simulink model "AD_model"  (R2025b)
settings: Solver=VariableStepAuto  StartTime=0.0  StopTime=tspan  RelTol=1e-3
values from neighbouring files (symbols this model uses):
  activado = 0    [run_AD_F.m]    (also in run_AD_s.m; run_AD_s_control.m)
  C_CO20 = 9    [AnaerobicDigestorParameters.m]
  C_CO2Din = 0    [AnaerobicDigestorParameters.m]
  C_HCO3in = 0    [AnaerobicDigestorParameters.m]
  F1 = 1    [run_AD_F.m]    (also in run_AD_s.m; run_AD_s_control.m)
  F2 = F2jumps(i)    [run_AD_F.m]    (also in run_AD_s.m = 1; run_AD_s_control.m = 1)
  K1 = 6.5e-7    (= 6.5e-07)    [AnaerobicDigestorParameters.m]
  KH = 3.25e-2    (= 0.0325)    [AnaerobicDigestorParameters.m]
  Ki = 0.667    [AnaerobicDigestorParameters.m]
  kLa = 100    [AnaerobicDigestorParameters.m]
  Ks = 0.0333    [AnaerobicDigestorParameters.m]
  mumax = 0.4    [AnaerobicDigestorParameters.m]
  P = 760    [AnaerobicDigestorParameters.m]
  P_CO20 = 273    [AnaerobicDigestorParameters.m]
  pHoff = 7    [AnaerobicDigestorParameters.m]
  pHth1 = 6.75    [AnaerobicDigestorParameters.m]
  pHth2 = 6.65    [AnaerobicDigestorParameters.m]
  pKa = 4.5    [AnaerobicDigestorParameters.m]
  QR1 = 50    [AnaerobicDigestorParameters.m]
  QR2 = 175    [AnaerobicDigestorParameters.m]
  rhoG = 38.9    [AnaerobicDigestorParameters.m]
  s0 = 2    [AnaerobicDigestorParameters.m]
  sif1 = 167    [run_AD_F.m]    (also in run_AD_s.m; run_AD_s_control.m)
  sif2 = sif1    (= 167)    [run_AD_F.m]    (also in run_AD_s.m = sifjumps(2); run_AD_s_control.m = sifjumps(i))
  V = 10    [AnaerobicDigestorParameters.m]
  VG = 2.0    (= 2)    [AnaerobicDigestorParameters.m]
  x0 = 5.28    [AnaerobicDigestorParameters.m]
  xin = 0    [AnaerobicDigestorParameters.m]
  Ych4x = 28.8    [AnaerobicDigestorParameters.m]
  Yco2x = 28.8    [AnaerobicDigestorParameters.m]
  Yxs = 0.032    [AnaerobicDigestorParameters.m]
  z0 = 50    [AnaerobicDigestorParameters.m]
  zin = 50    [AnaerobicDigestorParameters.m]
settings Model: Creator=Rodolfo  LastModifiedBy=Rodolfo

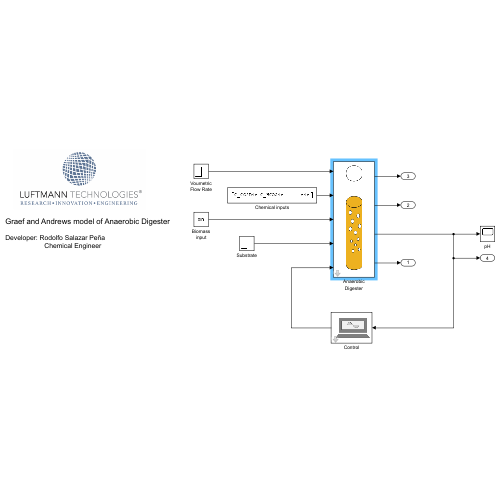
[thumbnail: Simulink's stored preview of the top-level diagram]
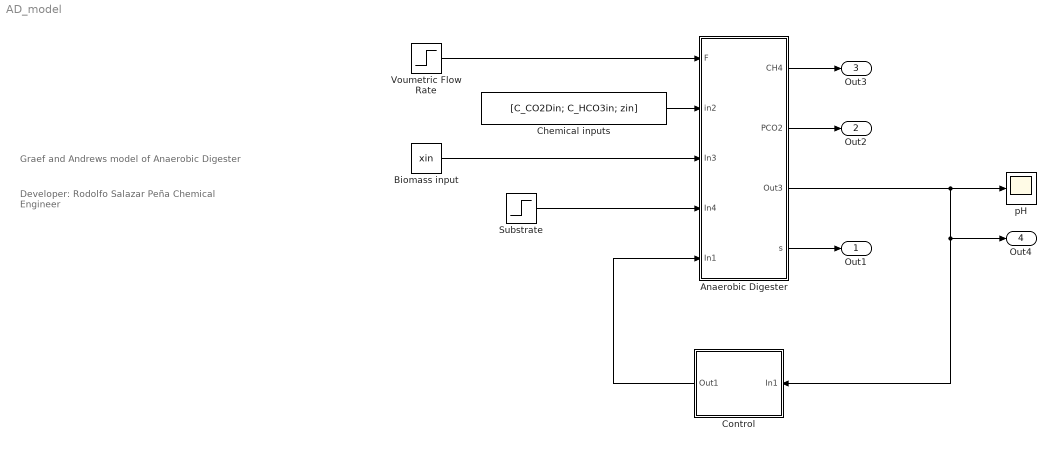
== system AD_model ==
  note: Developer: Rodolfo Salazar Peña
      | Chemical Engineer
  note: Graef and Andrews model of Anaerobic Digester
  Anaerobic Digester : Subsystem  mask(Anerobic Digester){VolumeParameter=V}
      mask prompts: VolumeParameter "Anarobic Digestor Volume"
      mask help: Integrated anaerobic digester model based on Graef and Andrews, combining biological, liquid, and gas phases for simulation and pH-oriented control studies.
      mask Help: This masked subsystem represents a complete anaerobic digester based on the Graef and Andrews model, integrating the biological, liquid, and gas phases into a unified dynamic framework. The biological phase describes the interaction between a generalized biomass and substrate using Haldane-type kinetics, accounting for substrate inhibition and biogas generation. The liquid phase models dissolved carbon dioxide and volatile fatty acids through chemical equilibria and gas–liquid mass transfer processes, enabling the determination and monitoring of pH to assess process stability and prevent acidification. The gas phase represents biogas release and composition, mainly methane and carbon dioxide, together with water vapor, hydrogen, and trace compounds, and supports control strategies based on gas manipulation, including the injection of inert compounds. This integrated model is intended for simulation, analysis, and control-oriented studies of anaerobic digestion systems.
  Biomass input : Constant  Value=xin
  Chemical inputs : Constant  Value=[C_CO2Din; C_HCO3in; zin]
  Control : Subsystem  mask(Control System){pHThreshold1=pHth1, pHThreshold2=pHth2, pHTurnedOff=pHoff, GasFlow1=QR1, GasFlow2=QR2}
      mask prompts: pHThreshold1 "pH Threshold 1"; pHThreshold2 "pH Threshold 2"; pHTurnedOff "pH off"; GasFlow1 "Volumetric Gas Flow Rate 1"; GasFlow2 "Volumetric Gas Flow Rate 2"
      mask help: Implements a two-stage relay control strategy based on pH monitoring to activate gas pumping and prevent acidification.
      mask Help: This masked subsystem implements a pH-based control strategy for the anaerobic digester. The pH of the liquid phase is continuously monitored and used as the controlled variable. Two relay elements with different threshold values define a staged control action. When the first pH threshold is reached, the first relay is activated, initiating gas pumping to mitigate acidification. If this action is insufficient and the pH continues to decrease until the second threshold is reached, a second relay is activated to increase the gas pumping rate. Once the pH returns to a neutral range, the activated pumps are deactivated. This subsystem is intended for dynamic simulation and evaluation of gas-based control strategies for acidification prevention.
      mask DialogControl pHParameterGroupVar Prompt: pH settings
      mask DialogControl GasFlows Prompt: Gas flow rates
  Substrate : Step  Before=sif1  After=sif2  SampleTime=0
  Voumetric Flow Rate : Step  Before=F1  After=F2  SampleTime=0
  pH : Scope
      settings: ActiveDisplayYMinimum=3.560384025804944  ActiveDisplayYMaximum=7.2867188541254588
  Out1 : Outport
  Out2 : Outport  Port=2
  Out3 : Outport  Port=3
  Out4 : Outport  Port=4
  wires:
  Chemical inputs/1 -> Anaerobic Digester/2(in2)
  Biomass input/1 -> Anaerobic Digester/3(In3)
  Substrate/1 -> Anaerobic Digester/4(In4)
  Anaerobic Digester/1(CH4) -> Out3/1
  Anaerobic Digester/2(PCO2) -> Out2/1
  Anaerobic Digester/4(s) -> Out1/1
  Anaerobic Digester/3(Out3) -> Control/1(In1), Out4/1, pH/1
  Voumetric Flow Rate/1 -> Anaerobic Digester/1(F)
  Control/1(Out1) -> Anaerobic Digester/5(In1)

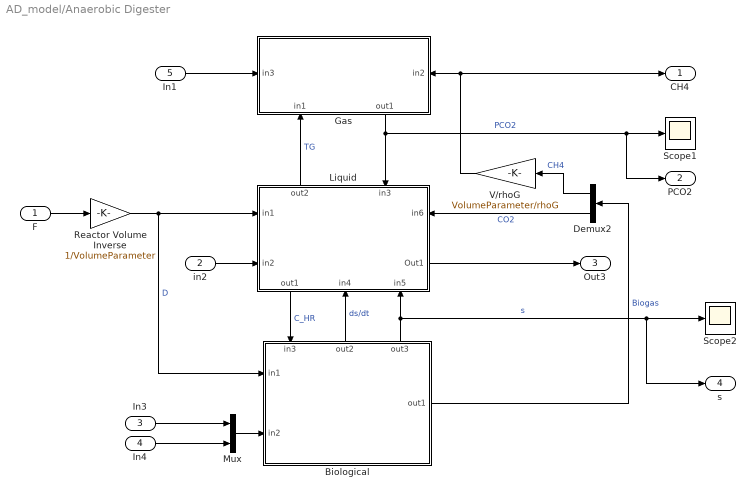
== system AD_model/Anaerobic Digester ==
  F : Inport
  in2 : Inport  Port=2
  In3 : Inport  Port=3
  In4 : Inport  Port=4
  In1 : Inport  Port=5
  Biological : Subsystem  Description=Image Credit: “Colorful Microorganisms: A Fascinating World Revealed” — image generated by Easy-Peasy.AI, licensed under Creative Commons. Source: easy-peasy.ai (https://easy-peasy.ai/ai-image-generator/images/colorful-microorganisms-intricate-shapes-forms-microbial-world  mask(Biological Phase){KinParameter1=mumax, KinParameter2=Ks, KinParameter3=Ki, YXS=Yxs, YCH4X=Ych4x, YCO2X=Yco2x, initx=x0, inits=s0}
      mask prompts: KinParameter1 "mu_max"; KinParameter2 "Ks"; KinParameter3 "Ki"; YXS "Y_x/s"; YCH4X "Y_CH4/x"; YCO2X "Y_CO2/x"; initx "x_0"; inits "s_0"
      mask help: Models the biological phase of an anaerobic digester with generalized biomass and substrate, using Haldane kinetics and biogas production (CH_4, CO_2).
      settings: PortSchema="{\"entries\":[{\"content\":{\"sides\":[{\"content\":{\"connectorIds\":[\"In1\",\"In2\"]},\"type\":\"ConnectorPlacement.EquallySpacedRectSide\",\"uuid\":\"94ecfc72-442c-41e1-8615-bec035df41b7\"},{\"content\":{\"connectorIds\":[\"Out1\"],\"side\":\"RIGHT\"},\"type\":\"ConnectorPlacement.EquallySpacedRectSide\",\"uuid\":\"bdca07f7-8c82-4860-9473-7970328f5f38\"},{\"content\":{\"connectorIds\":[\"In3\",\"Out2\",\"Out3\"],\"side\":\"TOP\"},\"type\":\"ConnectorPlacement.EquallySpacedRectSide\",\"uuid\":\"75f8fbf8-3bf9-45f3-a218-a686b6add209\"}]},\"type\":\"ConnectorPlacement.EquallySpacedConnector\",\"uuid\":\"e7f3f234-c871-423f-9938-c4e26176119c\"}],\"packageUris\":[\"http://schema.mathworks.com/mf0/Connector/R2020b\"],\"version\":\"1.0\"}"
      mask Help: This subsystem represents the biological phase of an anaerobic digester, describing the interaction between a generalized biomass 𝑥 and a substrate 𝑠. Microbial growth and substrate consumption are modeled using Haldane-type kinetics to account for substrate inhibition at high concentrations. Biogas production is computed as a consequence of the biological conversion process, with methane (CH_4) and carbon dioxide (CO_2) considered as the main gaseous products. The subsystem is intended for dynamic simulation and control-oriented analysis of anaerobic digestion processes.
      mask DialogControl KinParameterGroupVar Prompt: Kinetic Parameters
      mask DialogControl YieldsParameterGroupVar Prompt: Yields
      mask DialogControl InitialBio Prompt: Initial Conditions for Biological Phase
  Demux2 : Demux  Outputs=2
  Gas : Subsystem  Description=Image Credit: “Particle Model of a Gas (Teilchenmodell Gas)” — by Kaneiderdaniel, licensed under CC BY-SA 3.0. Source: Wikimedia Commons (File:Teilchenmodell_Gas.svg)  mask(Gas Phase){GasParameter1=P, GasParameter2=VG, GasParameter3=rhoG, InitGas=P_CO20}
      mask prompts: GasParameter1 "Pressure"; GasParameter2 "Gas Volume"; GasParameter3 "Gas Molar Density"; InitGas "CO2 Initial Partial Pressure"
      mask help: Models the gas phase of an anaerobic digester, including biogas release, composition dynamics, and gas-based control strategies to prevent acidification.
      settings: PortSchema="{\"entries\":[{\"content\":{\"sides\":[{\"content\":{\"connectorIds\":[\"In1\"]},\"type\":\"ConnectorPlacement.EquallySpacedRectSide\",\"uuid\":\"3565c727-b36c-46d2-95bd-ab32174b37cb\"},{\"content\":{\"connectorIds\":[\"In3\"],\"side\":\"RIGHT\"},\"type\":\"ConnectorPlacement.EquallySpacedRectSide\",\"uuid\":\"c4e665d1-7db3-4509-b4b2-58bd1ad74d47\"},{\"content\":{\"side\":\"TOP\"},\"type\":\"ConnectorPlacement.EquallySpacedRectSide\",\"uuid\":\"7f169c89-e67a-49df-a15c-98b353f69781\"},{\"content\":{\"connectorIds\":[\"In2\",\"Out1\"],\"side\":\"BOTTOM\"},\"type\":\"ConnectorPlacement.EquallySpacedRectSide\",\"uuid\":\"61ad4f32-0a2a-4148-a498-3c1351082a85\"}]},\"type\":\"ConnectorPlacement.EquallySpacedConnector\",\"uuid\":\"c5dc36fd-dcdd-47be-95df-e8a0ac72026a\"}],\"packageUris\":[\"http://schema.mathworks.com/mf0/Connector/R2020b\"],\"version\":\"1.0\"}"
      mask Help: This masked subsystem represents the gas phase of an anaerobic digester, where biogas is released as a result of biological conversion processes. The biogas is composed mainly of methane and carbon dioxide, along with water vapor, molecular hydrogen and trace compounds. The gas phase plays a key role in process operation and control, since acidification prevention strategies may involve the injection or removal of inert gases to influence gas composition, partial pressures, and gas–liquid equilibria. This subsystem is intended for dynamic simulation and control-oriented analysis of the anaerobic digestion process.
      mask DialogControl GasParameterGroupVar Prompt: Gas Parameters
      mask DialogControl GasInit Prompt: Gas Initial Conditions
  Liquid : Subsystem  Description=Image Credit: “Liquid Water Waves Background” — image by Andrea Stöckel, in the public domain (CC0). Source: PublicDomainPictures.net (https://www.publicdomainpictures.net/es/view-image.php?image=431076&picture=liquido-de-fondo-de-agua-de-ondas)  mask(Liquid phase of an anaerobic digester){TGParameter1=KH, TGParameter2=kLa, IonParameter1=pKa, IonParameter2=K1, InitLiquid1=C_CO20, InitLiquid2=z0}
      mask prompts: TGParameter1 "Henry's Law constant"; TGParameter2 "Bulk - Interphase constnat"; IonParameter1 "VFA Dissociation"; IonParameter2 "Dissolved CO2 Equilibrium"; InitLiquid1 "Dissolved CO2 Initial Concentration"; InitLiquid2 "Net Cationic Initial Concentration"
      mask help: Models liquid-phase chemistry and mass transfer in an anaerobic digester to compute and monitor pH and prevent acidification.
      settings: PortSchema="{\"entries\":[{\"content\":{\"sides\":[{\"content\":{\"connectorIds\":[\"In1\",\"In2\"]},\"type\":\"ConnectorPlacement.EquallySpacedRectSide\",\"uuid\":\"2cd52875-f219-461b-bc38-0fc8a9bb25f3\"},{\"content\":{\"connectorIds\":[\"In6\",\"Out1\"],\"side\":\"RIGHT\"},\"type\":\"ConnectorPlacement.EquallySpacedRectSide\",\"uuid\":\"4617526c-ef4d-41e9-b20c-a88def61ea23\"},{\"content\":{\"connectorIds\":[\"Out3\",\"In3\"],\"side\":\"TOP\"},\"type\":\"ConnectorPlacement.EquallySpacedRectSide\",\"uuid\":\"65a01b26-7f6a-43a7-a50c-408a5bf6dc68\"},{\"content\":{\"connectorIds\":[\"Out2\",\"In4\",\"In5\"],\"side\":\"BOTTOM\"},\"type\":\"ConnectorPlacement.EquallySpacedRectSide\",\"uuid\":\"34e478b9-109e-4b95-ae18-09426b257fdc\"}]},\"type\":\"ConnectorPlacement.EquallySpacedConnector\",\"uuid\":\"457643e1-ae11-400d-8d76-b246d90ceafd\"}],\"packageUris\":[\"http://schema.mathworks.com/mf0/Connector/R2020b\"],\"version\":\"1.0\"}"
      mask Help: This masked subsystem represents the liquid phase of an anaerobic digester, where dissolved carbon dioxide and volatile fatty acids (VFAs) undergo chemical equilibria and mass transfer processes. The model accounts for acid–base reactions, dissociation phenomena, and gas–liquid mass transfer effects that influence the hydrogen ion concentration. The primary objective of this subsystem is to determine and monitor the pH of the liquid phase in order to assess process stability and prevent acidification during anaerobic digestion.
      mask DialogControl TransferParameterGroupVar Prompt: Transfer CO2 gas - liquid
      mask DialogControl IonicParameters Prompt: Ionics Equilibriums
      mask DialogControl InitiLiquid Prompt: Initial Conditions for Liquid Phase
  Mux : Mux  Inputs=2
  Reactor Volume Inverse : Gain  Gain=1/VolumeParameter
  Scope1 : Scope
      settings: ActiveDisplayYMinimum=-1  ActiveDisplayYMaximum=1
  Scope2 : Scope
      settings: ActiveDisplayYMinimum=-1  ActiveDisplayYMaximum=1  DataLoggingVariableName=ScopeData2
  V/rhoG : Gain  Gain=VolumeParameter/rhoG
  CH4 : Outport
  PCO2 : Outport  Port=2
  Out3 : Outport  Port=3
  s : Outport  Port=4
  wires:
  Biological/2(out2) -> Liquid/4(in4)  "ds/dt"
  Liquid/2(out1) -> Biological/3(in3)  "C_HR"
  Liquid/3(out2) -> Gas/2(in1)  "TG"
  Biological/1(out1) -> Demux2/1  "Biogas"
  Biological/3(out3) -> Liquid/5(in5), s/1, Scope2/1  "s"
  Demux2/2 -> Liquid/6(in6)  "CO2"
  Gas/1(out1) -> Liquid/3(in3), PCO2/1, Scope1/1  "PCO2"
  F/1 -> Reactor Volume Inverse/1
  Mux/1 -> Biological/2(in2)
  Demux2/1 -> V/rhoG/1  "CH4"
  In3/1 -> Mux/1
  Liquid/1(Out1) -> Out3/1
  in2/1 -> Liquid/2(in2)
  In4/1 -> Mux/2
  In1/1 -> Gas/1(in3)
  V/rhoG/1 -> Gas/3(in2), CH4/1
  Reactor Volume Inverse/1 -> Biological/1(in1), Liquid/1(in1)  "D"

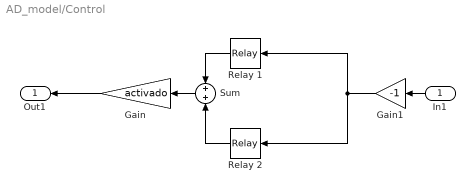
== system AD_model/Control ==
  In1 : Inport
  Gain : Gain  Gain=activado
  Gain1 : Gain  Gain=-1
  Relay 1 : Relay  OnSwitchValue=-pHThreshold1  OffSwitchValue=-pHTurnedOff  OnOutputValue=GasFlow1
  Relay 2 : Relay  OnSwitchValue=-pHThreshold2  OffSwitchValue=-pHTurnedOff  OnOutputValue=GasFlow2
  Sum : Sum
  Out1 : Outport
  wires:
  Relay 1/1 -> Sum/1
  In1/1 -> Gain1/1
  Relay 2/1 -> Sum/2
  Gain/1 -> Out1/1
  Sum/1 -> Gain/1
  Gain1/1 -> Relay 1/1, Relay 2/1

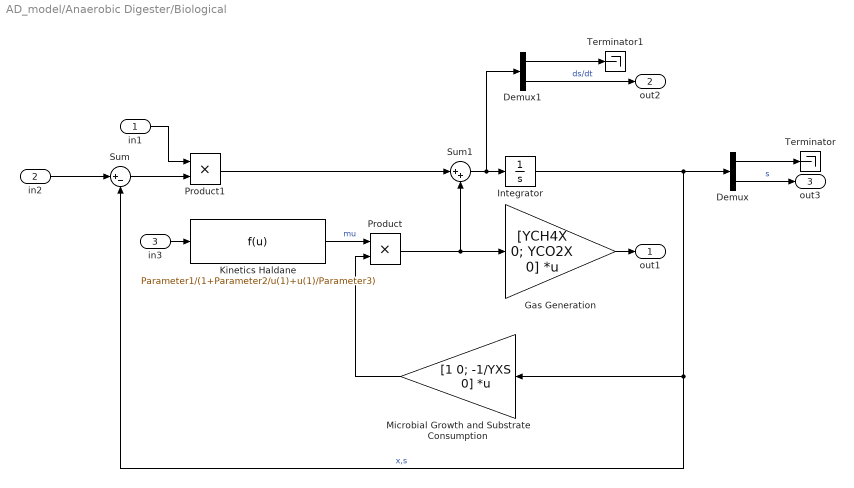
== system AD_model/Anaerobic Digester/Biological ==
  in1 : Inport
  in2 : Inport  Port=2
  in3 : Inport  Port=3
  Demux : Demux  Outputs=2
  Demux1 : Demux  Outputs=2
  Gas Generation : Gain  Gain=[YCH4X 0; YCO2X 0]  Multiplication=Matrix(K*u)
  Integrator : Integrator  InitialCondition=[initx; inits]
  Kinetics Haldane : Fcn  Expr=Parameter1/(1+Parameter2/u(1)+u(1)/Parameter3)  mask(Biochemical Kinetics){Parameter1=KinParameter1, Parameter2=KinParameter2, Parameter3=KinParameter3}
      mask prompts: Parameter1 "Maximal Specific Growth"; Parameter2 "Saturation"; Parameter3 "Inhibition"
      mask help: Models substrate-inhibited reaction kinetics using the Haldane formulation, suitable for biochemical and microbial process simulations.
      mask Help:
      | This block implements Haldane-type biochemical kinetics to model substrate-inhibited reaction rates. The reaction rate follows a modified Monod formulation that accounts for inhibitory effects at high substrate concentrations. This model is commonly used to describe microbial growth or enzymatic reactions where excess substrate reduces the overall reaction rate. The block computes the reaction rate as a function of substrate concentration and kinetic parameters, and is intended for dynamic simulation, analysis, and control-oriented studies of biochemical processes.
      | 
      | \[
      | \mu=
      | \]
  Microbial Growth and Substrate Consumption : Gain  Gain=[1 0; -1/YXS 0]  Multiplication=Matrix(K*u)
  Product : Product
  Product1 : Product
  Sum : Sum  Inputs=|+-
  Sum1 : Sum  Inputs=|++
  Terminator : Terminator
  Terminator1 : Terminator
  out1 : Outport
  out2 : Outport  Port=2
  out3 : Outport  Port=3
  wires:
  Integrator/1 -> Demux/1, Microbial Growth and Substrate Consumption/1, Sum/2  "x,s"
  Microbial Growth and Substrate Consumption/1 -> Product/2
  Kinetics Haldane/1 -> Product/1  "mu"
  in2/1 -> Sum/1
  Sum/1 -> Product1/2
  in1/1 -> Product1/1
  in3/1 -> Kinetics Haldane/1
  Product1/1 -> Sum1/1
  Sum1/1 -> Demux1/1, Integrator/1
  Product/1 -> Sum1/2, Gas Generation/1
  Demux/1 -> Terminator/1
  Demux/2 -> out3/1  "s"
  Demux1/2 -> out2/1  "ds/dt"
  Demux1/1 -> Terminator1/1
  Gas Generation/1 -> out1/1

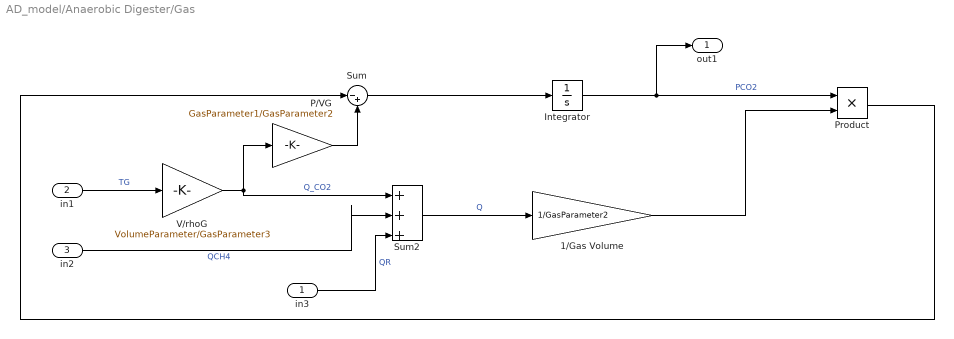
== system AD_model/Anaerobic Digester/Gas ==
  in3 : Inport
  in1 : Inport  Port=2
  in2 : Inport  Port=3
  1/Gas Volume : Gain  Gain=1/GasParameter2
  Integrator : Integrator  InitialCondition=InitGas
  P/VG : Gain  Gain=GasParameter1/GasParameter2
  Product : Product
  Sum : Sum  Inputs=|-+
  Sum2 : Sum  Inputs=++|+
  V/rhoG : Gain  Gain=VolumeParameter/GasParameter3
  out1 : Outport
  wires:
  Sum/1 -> Integrator/1
  Integrator/1 -> out1/1, Product/1  "PCO2"
  Product/1 -> Sum/1
  in1/1 -> V/rhoG/1  "TG"
  in2/1 -> Sum2/2  "QCH4"
  Sum2/1 -> 1/Gas Volume/1  "Q"
  V/rhoG/1 -> P/VG/1, Sum2/1  "Q_CO2"
  in3/1 -> Sum2/3  "QR"
  P/VG/1 -> Sum/2
  1/Gas Volume/1 -> Product/2

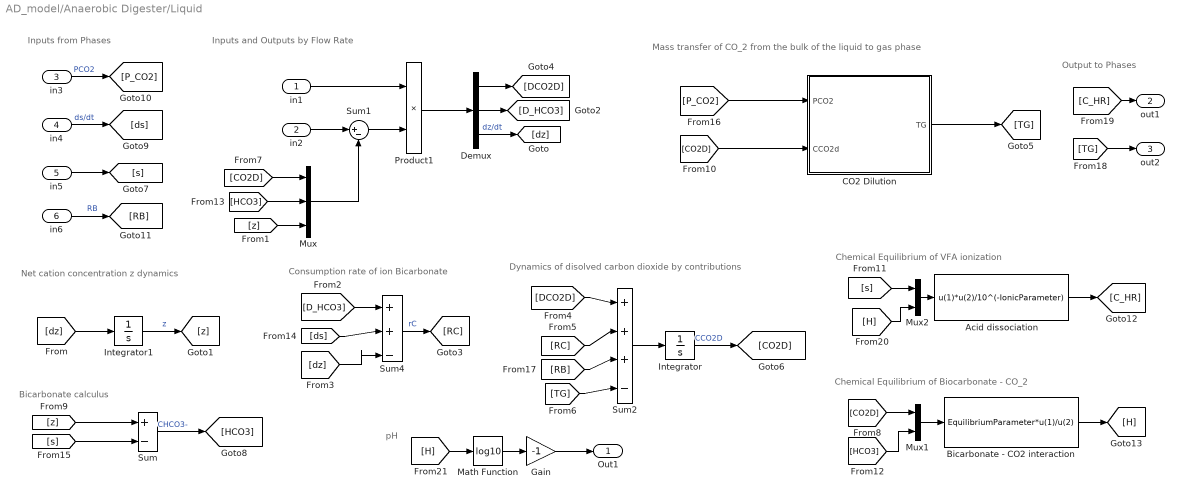
== system AD_model/Anaerobic Digester/Liquid ==
  note: pH
  note: Chemical Equilibrium of Biocarbonate - CO_2
  note: Chemical Equilibrium of VFA ionization
  note: Output to Phases
  note: Mass transfer of CO_2 from the bulk of the liquid to gas phase
  note: Bicarbonate calculus
  note: Inputs and Outputs by Flow Rate
  note: Inputs from Phases
  note: Dynamics of disolved carbon dioxide by contributions
  note: Consumption rate of ion Bicarbonate
  note: Net cation concentration z dynamics
  in1 : Inport
  in2 : Inport  Port=2
  in3 : Inport  Port=3
  in4 : Inport  Port=4
  in5 : Inport  Port=5
  in6 : Inport  Port=6
  Acid dissociation : Fcn  Expr=u(1)*u(2)/10^(-IonicParameter)  mask(VFAs Ionic Equilibrium){IonicParameter=IonParameter1}
      mask prompts: IonicParameter "Dissociation Ionic Constant"
      mask help: Models the ionic equilibrium of VFAs using pKa.
      mask Help: This block calculates the dissociation of VFAs in the liquid phase. This equilibrium is modeled using the dissociation constant expressed as pKa, allowing the equilibrium concentrations of the ionic species to be determined as a function of ion hydrogen dissolved. This block is intended for dynamic simulation of pH-related phenomena and carbonate chemistry in anaerobic digestion and other biochemical systems.
  Bicarbonate - CO2 interaction : Fcn  Expr=EquilibriumParameter*u(1)/u(2)  mask(Carbon Dioxide Ionic Equilibrium){EquilibriumParameter=IonParameter2}
      mask prompts: EquilibriumParameter "Equilibrium Constant"
      mask help: Models the dissociation of dissolved carbon dioxide into ion hydrogen and ion bicarbonate.
      mask Help: This block calculates the dissociation of dissolved carbon dioxide in the liquid phase into hydrogen ions and bicarbonate ions. The acid–base equilibrium is modeled using the dissociation constant expressed as K1, allowing the equilibrium concentrations of the ionic species to be determined as a function of dissolved carbon dioxide. This block is intended for dynamic simulation of pH-related phenomena and carbonate chemistry in anaerobic digestion and other biochemical systems.
  CO2 Dilution : Subsystem
  Demux : Demux  Outputs=3
  Gain : Gain  Gain=-1
  Integrator : Integrator  InitialCondition=InitLiquid1
  Integrator1 : Integrator  InitialCondition=InitLiquid2
  Math Function : Math  Operator=log10
  Mux : Mux  Inputs=3
  Mux1 : Mux  Inputs=2
  Mux2 : Mux  Inputs=2
  Product1 : Product
  Sum : Sum  Inputs=+-
  Sum1 : Sum  Inputs=|+-
  Sum2 : Sum  Inputs=+|++-
  Sum4 : Sum  Inputs=+|+-
  Out1 : Outport
  out1 : Outport  Port=2
  out2 : Outport  Port=3
  wires:
  in1/1 -> Product1/1
  in2/1 -> Sum1/1
  Sum1/1 -> Product1/2
  Product1/1 -> Demux/1
  Mux2/1 -> Acid dissociation/1
  CO2 Dilution/1(TG) -> [TG]
  Mux/1 -> Sum1/2
  Integrator1/1 -> [z]  "z"
  Demux/3 -> [dz]  "dz/dt"
  [dz] -> Integrator1/1
  [z] -> Mux/3
  [D_HCO3] -> Sum4/1
  Demux/2 -> [D_HCO3]
  [dz] -> Sum4/3
  Sum4/1 -> [RC]  "rC"
  Demux/1 -> [DCO2D]
  [DCO2D] -> Sum2/1
  Sum2/1 -> Integrator/1
  Integrator/1 -> [CO2D]  "CCO2D"
  [CO2D] -> Mux/1
  [CO2D] -> Mux1/1
  Mux1/1 -> Bicarbonate - CO2 interaction/1
  [z] -> Sum/1
  [CO2D] -> CO2 Dilution/2(CCO2d)
  [s] -> Mux2/1
  Sum/1 -> [HCO3]  "CHCO3-"
  [HCO3] -> Mux1/2
  [HCO3] -> Mux/2
  in4/1 -> [ds]  "ds/dt"
  [ds] -> Sum4/2
  in5/1 -> [s]
  [s] -> Sum/2
  in3/1 -> [P_CO2]  "PCO2"
  [P_CO2] -> CO2 Dilution/1(PCO2)
  in6/1 -> [RB]  "RB"
  Acid dissociation/1 -> [C_HR]
  [TG] -> out2/1
  [C_HR] -> out1/1
  Bicarbonate - CO2 interaction/1 -> [H]
  [H] -> Mux2/2
  [H] -> Math Function/1
  Math Function/1 -> Gain/1
  Gain/1 -> Out1/1
  [RC] -> Sum2/2
  [RB] -> Sum2/3
  [TG] -> Sum2/4

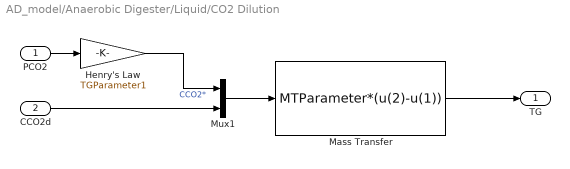
== system AD_model/Anaerobic Digester/Liquid/CO2 Dilution ==
  PCO2 : Inport
  CCO2d : Inport  Port=2
  Henry's Law : Gain  Gain=TGParameter1
  Mass Transfer : Fcn  Expr=MTParameter*(u(2)-u(1))  mask(Mass transfer of carbon dioxide from bulk liquid to interphase){MTParameter=TGParameter2}
      mask prompts: MTParameter "Mass Transfer Coefficient"
      mask help: Computes CO_2 mass transfer from liquid bulk to the gas–liquid interface using a kLa formulation.
      mask Help: This block computes the mass transfer of carbon dioxide from the bulk liquid phase to the gas–liquid interface. The transfer rate is modeled using a volumetric mass transfer coefficient kLa, which accounts for both the liquid-side mass transfer coefficient and the effective interfacial area. The driving force for mass transfer is defined by the difference between the bulk liquid CO_2 concentration and its equilibrium concentration at the gas–liquid interface. This block is intended for dynamic simulation of gas–liquid mass transfer phenomena in biochemical and anaerobic digestion systems.
  Mux1 : Mux  Inputs=2
  TG : Outport
  wires:
  Henry's Law/1 -> Mux1/1  "CCO2*"
  CCO2d/1 -> Mux1/2
  PCO2/1 -> Henry's Law/1
  Mux1/1 -> Mass Transfer/1
  Mass Transfer/1 -> TG/1
